simulink model "Suspension"  (R2023b)
settings: Solver=VariableStepAuto  StartTime=0.0  StopTime=50  RelTol=1e-3
values from neighbouring files (symbols this model uses):
  b1 = 350    [Suspension_Model_parameters.m]
  b2 = 15020    [Suspension_Model_parameters.m]
  k1 = 80000    [Suspension_Model_parameters.m]
  k2 = 500000    [Suspension_Model_parameters.m]
  m1 = 2500    [Suspension_Model_parameters.m]
  m2 = 320    [Suspension_Model_parameters.m]
settings Model: Creator=mdhel  LastModifiedBy=mdhel

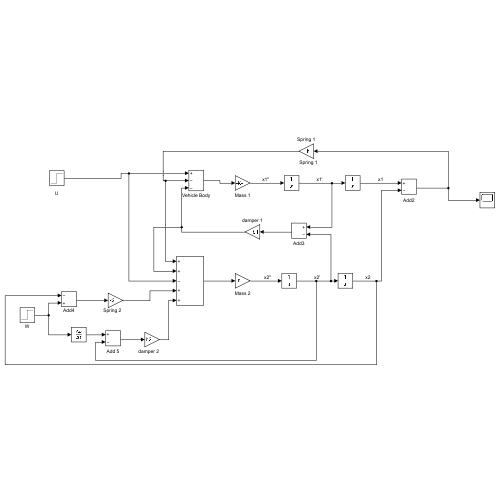
[thumbnail: Simulink's stored preview of the top-level diagram]
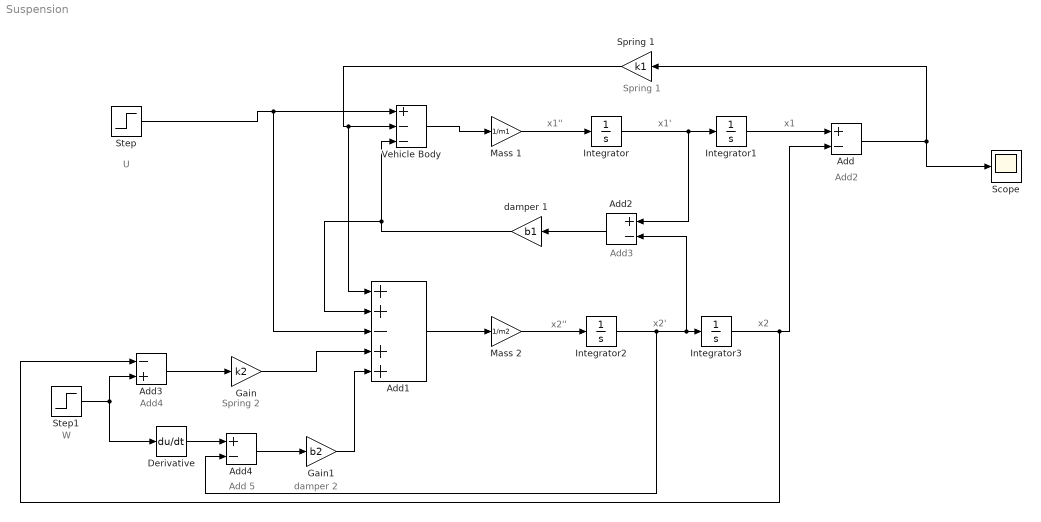
== system Suspension ==
  note: W
  note: damper 2
  note: Add 5
  note: Spring 1
  note: Spring 2
  note: Add4
  note: Add2
  note: Add3
  note: U
  note: x2
  note: x2'
  note: x2''
  note: x1
  note: x1'
  note: x1''
  Add : Sum  Inputs=+-
  Add1 : Sum  Inputs=++-++
  Add2 : Sum  Inputs=+-
  Add3 : Sum  Inputs=-+
  Add4 : Sum  Inputs=+-
  Derivative : Derivative
  Gain : Gain  Gain=k2
  Gain1 : Gain  Gain=b2
  Integrator{,1..3} (4 alike) : Integrator
  Mass 1 : Gain  Gain=1/m1
  Mass 2 : Gain  Gain=1/m2
  Scope : Scope
  Spring 1 : Gain  Gain=k1
  Step : Step  SampleTime=0
  Step1 : Step  After=0  SampleTime=0
  Vehicle Body : Sum  Inputs=+--
  damper 1 : Gain  Gain=b1
  wires:
  Step/1 -> Add1/3, Vehicle Body/1
  Vehicle Body/1 -> Mass 1/1
  Mass 1/1 -> Integrator/1
  Integrator/1 -> Add2/1, Integrator1/1
  Integrator1/1 -> Add/1
  Add/1 -> Spring 1/1, Scope/1
  Spring 1/1 -> Add1/1, Vehicle Body/2
  Add1/1 -> Mass 2/1
  Mass 2/1 -> Integrator2/1
  Integrator3/1 -> Add3/1, Add/2
  Integrator2/1 -> Add4/2, Add2/2, Integrator3/1
  Add2/1 -> damper 1/1
  damper 1/1 -> Add1/2, Vehicle Body/3
  Step1/1 -> Add3/2, Derivative/1
  Add3/1 -> Gain/1
  Gain/1 -> Add1/4
  Derivative/1 -> Add4/1
  Add4/1 -> Gain1/1
  Gain1/1 -> Add1/5
